simulink model "statisticalAttitude"  (R2023b)
settings: Solver=VariableStepAuto  StartTime=0.0  StopTime=Tfinal  RelTol=1e-3
libraries: matrix_library x1, rotationConversionLib x1
settings Model: Creator=kristopherriordan  LastModifiedBy=kristopherriordan

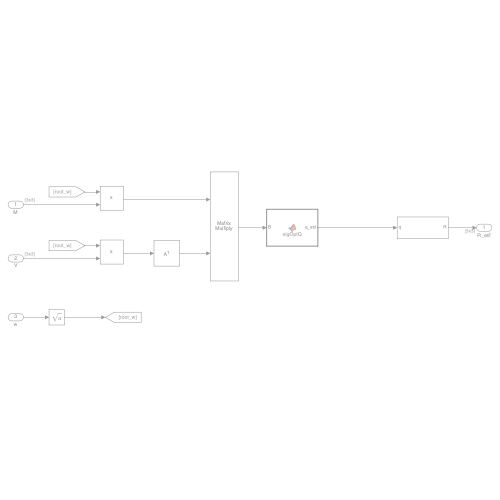
[thumbnail: Simulink's stored preview of the top-level diagram]
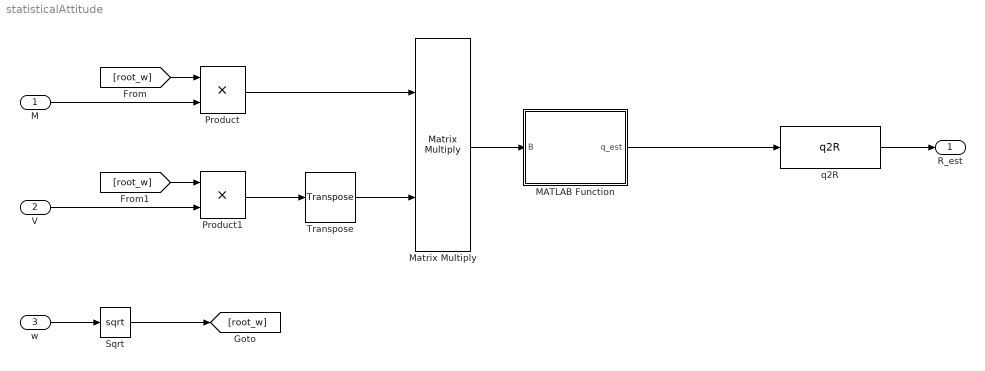
== system statisticalAttitude ==
  M : Inport  PortDimensions=[3 3]
  V : Inport  Port=2  PortDimensions=[3 3]
  w : Inport  Port=3
  MATLAB Function : MATLAB Function  TreatAsAtomicUnit=on
  Matrix Multiply : Product  Multiplication=Matrix(*)
  Product : Product
  Product1 : Product
  Sqrt : Sqrt
  Transpose : matrix_library/Transpose
  q2R : rotationConversionLib/q2R  SystemSampleTime=-1  VariantActivationTime=update diagram  AllowFlexibleInterface=on  Latency=0  AutoFrameSizeCalculation=off
  R_est : Outport  PortDimensions=[3 3]
  wires:
  w/1 -> Sqrt/1
  Sqrt/1 -> [root_w]
  [root_w] -> Product/1
  M/1 -> Product/2
  V/1 -> Product1/2
  [root_w] -> Product1/1
  Product/1 -> Matrix Multiply/1
  Product1/1 -> Transpose/1
  Transpose/1 -> Matrix Multiply/2
  Matrix Multiply/1 -> MATLAB Function/1(B)
  MATLAB Function/1(q_est) -> q2R/1
  q2R/1 -> R_est/1

== matlab function statisticalAttitude/MATLAB Function ==
  data: B input size=[3 3]; q_est output
function q_est = eigOptQ(B)

q_est = zeros([4 1]);

S = B + B.';

Z = [B(2,3) - B(3,2), B(3,1) - B(1,3), B(1,2) - B(2,1)].';

sig = trace(B);

K = [S - sig.*eye(3), Z;Z.', sig];

[V,D] = eig(K);

[~, idx] = max(diag(D));

q_est = V(:, idx);
